simulink model "PT_TrqRat"  (R2016b)
settings: configuration reference "CodeGenConfigSet" (kept outside this file)
values from neighbouring files (symbols this model uses):
  PT_rTrqDfl_C = Calibration.Parameter    [init_PT_TrqRat.m]    (also in init_PT_TrqRat_SIL.m = Simulink.Parameter)
  PT_rTrqMax_C = Calibration.Parameter    [init_PT_TrqRat.m]    (also in init_PT_TrqRat_SIL.m = Simulink.Parameter)
  PT_rTrqMin_C = Calibration.Parameter    [init_PT_TrqRat.m]    (also in init_PT_TrqRat_SIL.m = Simulink.Parameter)
  PT_swtDetTypeCAN_C = Calibration.Parameter    [init_PT_TrqRat.m]    (also in init_PT_TrqRat_SIL.m = Simulink.Parameter)
  PT_vMinTrqRat_C = Calibration.Parameter    [init_PT_TrqRat.m]    (also in init_PT_TrqRat_SIL.m = Simulink.Parameter)
undefined symbols (not defined in the file or in its folder): PT_TraType_State_conv, Switch_conv
libraries: CXLib x1
settings Model: Creator=Administrator  LastModifiedBy=lenovo
settings ConfigSetRef: SourceLocation=Base Workspace

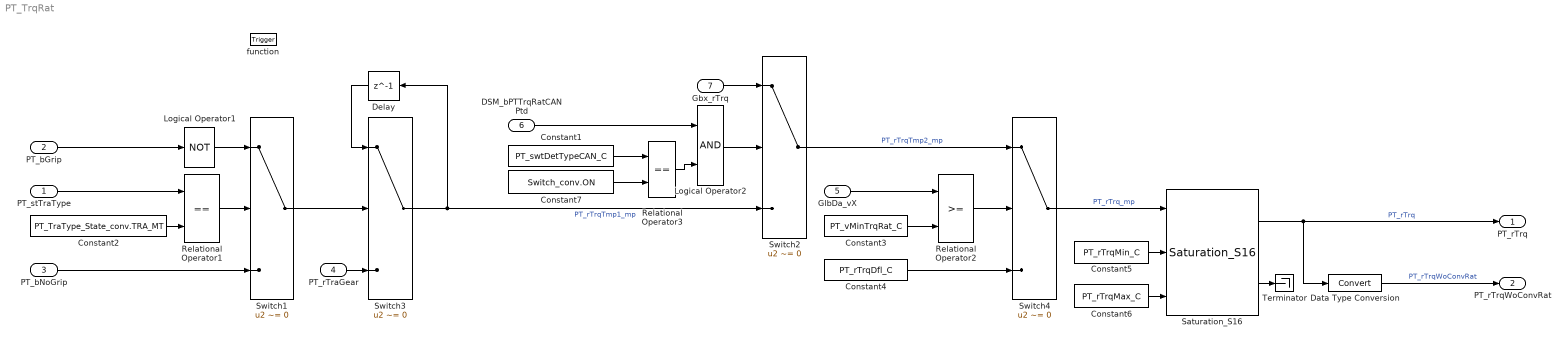
== system PT_TrqRat ==
  PT_stTraType : Inport  Description=Current transmission type  OutDataTypeStr=Enum: PT_TraType_State_conv
  PT_bGrip : Inport  Description=Grip is for sure present (the converter lockup clutch / the automated or manual clutch is completely closed and PT_bNoGrip = FALSE)  Port=2  OutMin=0  OutMax=1  OutDataTypeStr=boolean
  PT_bNoGrip : Inport  Description=Grip reliable exclude  Port=3  OutMin=0  OutMax=1  OutDataTypeStr=boolean
  PT_rTraGear : Inport  Description=Current ratio for transmission  Port=4  OutMin=-100  OutMax=100  OutDataTypeStr=TransRatio
  GlbDa_vX : Inport  Tag=km/h  Description=Longitudinal vehicle speed (X-direction)  Port=5  OutMin=0  OutMax=250  OutDataTypeStr=VehSpeed_km_h
  DSM_bPTTrqRatCANPtd : Inport  Description=status of FId_PTTrqRatCANPtd  Port=6  OutMin=0  OutMax=1  OutDataTypeStr=boolean
  Gbx_rTrq : Inport  Description=Transmission function information from Gearbox ECU(including Torque converter)  Port=7  OutMin=-100  OutMax=100  OutDataTypeStr=TransRatio
  function : TriggerPort  TriggerType=function-call  VariantControl=Variant
  Constant1 : Constant  RequirementInfo={} %GIDa_51935ed2_82be_46fc_9ec8_e95d2da59e17  Value=PT_swtDetTypeCAN_C
  Constant2 : Constant  RequirementInfo={'other' 'APP_requirements.doc' '@Simulink_requirement_item_25' 'true' '手动开关' '' } %GIDa_a24cac6a_9420_4488_8ae3_e922a0c48dc7  Value=PT_TraType_State_conv.TRA_MT
  Constant3 : Constant  RequirementInfo={'other' 'APP_requirements.doc' '@Simulink_requirement_item_25' 'true' '手动开关' '' } %GIDa_76b09556_6dfc_4f36_aba1_bcbeabbfb8b8  Value=PT_vMinTrqRat_C
  Constant4 : Constant  RequirementInfo={'other' 'APP_requirements.doc' '@Simulink_requirement_item_25' 'true' '手动开关' '' } %GIDa_fc5ffafe_4a99_42ab_bca6_2db6c09b2033  Value=PT_rTrqDfl_C
  Constant5 : Constant  RequirementInfo={'other' 'APP_requirements.doc' '@Simulink_requirement_item_25' 'true' '手动开关' '' } %GIDa_38c850e6_7f9d_43c7_8fe5_4b1a595cdf8e  Value=PT_rTrqMin_C
  Constant6 : Constant  RequirementInfo={'other' 'APP_requirements.doc' '@Simulink_requirement_item_25' 'true' '手动开关' '' } %GIDa_3f163217_6647_4ec2_a0ec_eebdd4ace4b3  Value=PT_rTrqMax_C
  Constant7 : Constant  RequirementInfo={} %GIDa_bd7ffad5_1f14_49f1_a9a7_6311ac5a8e1c  Value=Switch_conv.ON
  Data Type Conversion : DataTypeConversion
  Delay : Delay  DelayLength=1  InitialCondition=0
  Logical Operator1 : Logic  Operator=NOT  AllPortsSameDT=off  OutDataTypeStr=boolean
  Logical Operator2 : Logic  AllPortsSameDT=off  OutDataTypeStr=boolean
  Relational Operator1 : RelationalOperator  Operator===  OutDataTypeStr=boolean  RndMeth=Simplest  InputSameDT=on
  Relational Operator2 : RelationalOperator  OutDataTypeStr=boolean  RndMeth=Simplest  InputSameDT=on
  Relational Operator3 : RelationalOperator  Operator===  OutDataTypeStr=boolean  RndMeth=Simplest  InputSameDT=on
  Saturation_S16 : CXLib/Saturation_S16
  Switch1 : Switch  Criteria=u2 ~= 0  InputSameDT=on
  Switch2 : Switch  Criteria=u2 ~= 0  SaturateOnIntegerOverflow=on  InputSameDT=on
  Switch3 : Switch  Criteria=u2 ~= 0  InputSameDT=on
  Switch4 : Switch  Criteria=u2 ~= 0  InputSameDT=on
  Terminator : Terminator
  PT_rTrq : Outport  Description=Powertrain torque ratio  OutMin=-100  OutMax=100  OutDataTypeStr=TransRatio
  PT_rTrqWoConvRat : Outport  Description=torque ratio of the power train without differential and converter torque ratio  Port=2  OutMin=-100  OutMax=100  OutDataTypeStr=TransRatio
  wires:
  Saturation_S16/1 -> PT_rTrq/1, Data Type Conversion/1  "PT_rTrq"
  Constant6/1 -> Saturation_S16/3
  GlbDa_vX/1 -> Relational Operator2/1
  Constant4/1 -> Switch4/3
  Constant3/1 -> Relational Operator2/2
  PT_stTraType/1 -> Relational Operator1/1
  Constant2/1 -> Relational Operator1/2
  Switch1/1 -> Switch3/2
  Delay/1 -> Switch3/1
  PT_bGrip/1 -> Logical Operator1/1
  Logical Operator1/1 -> Switch1/1
  Relational Operator2/1 -> Switch4/2
  PT_bNoGrip/1 -> Switch1/3
  PT_rTraGear/1 -> Switch3/3
  Relational Operator1/1 -> Switch1/2
  Constant5/1 -> Saturation_S16/2
  Switch4/1 -> Saturation_S16/1  "PT_rTrq_mp"
  Saturation_S16/2 -> Terminator/1
  DSM_bPTTrqRatCANPtd/1 -> Logical Operator2/1
  Logical Operator2/1 -> Switch2/2
  Constant7/1 -> Relational Operator3/2
  Constant1/1 -> Relational Operator3/1
  Relational Operator3/1 -> Logical Operator2/2
  Gbx_rTrq/1 -> Switch2/1
  Switch3/1 -> Switch2/3, Delay/1  "PT_rTrqTmp1_mp"
  Data Type Conversion/1 -> PT_rTrqWoConvRat/1  "PT_rTrqWoConvRat"
  Switch2/1 -> Switch4/1  "PT_rTrqTmp2_mp"
